simulink model "H8_6GDL_lineal_modelo"  (R2022b)
settings: Solver=VariableStepAuto  StartTime=0.0  StopTime=5  MaxStep=1e-3  RelTol=1e-3
InitFcn:
  | cg_nom=0.567;
  | cg_suelo=0.56985;
  | cg_techo=0.54735;
values from neighbouring files (symbols this model uses):
  A6 = [0 0 0 0 0 0 0 0 0 0 0 0 ... (100 elements, 10x10)]    [matrices_linealizacion_6gdl.mat]
  B6 = [0 0 0 0 0 0.000575563603666 -0.0459993641186 -0.0505103975277 0.151580453785 0.00175830093621 0 0 ... (80 elements, 10x8)]    [matrices_linealizacion_6gdl.mat]
  C6 = [1 0 0 0 0 0 0 0 0 0 0 1 ... (100 elements, 10x10)]    [matrices_linealizacion_6gdl.mat]
  D6 = [0 0 0 0 0 0 0 0 0 0 0 0 ... (80 elements, 10x8)]    [matrices_linealizacion_6gdl.mat]
  Ka = [34.5916764023 4.46928641015 34.7816336405 4.65924364837 92.2484067139 -92.2484067139 74.2332308826 -74.2332308826 -4220.94514487 -4209.6309051 -4205.06787146 -4193.7536317 ... (120 elements, 8x15)]    [Ka.mat]    (also in linealizacion_5gdl_bien.m = place(Aa,Ba,[ -1.5 -1.5 -1.5 -1.5 -2 -2 -6 -6 -7 -7 -5 -5 -2; linealizacion_EMS.m = place(Aa,Ba,[ -1 -1 -2 -2 -3 -3 -6 -6 -7 -7 -5 -5 -4 -4 -5 -)
undefined symbols (not defined in the file or in its folder): ems, hems, magnitude
libraries: simulink x5
settings Model: Creator=aceao  LastModifiedBy=USUARIO
settings SolverCC: ZeroCrossAlgorithm=Adaptive
settings DebuggingCC: IgnoredZcDiagnostic=none

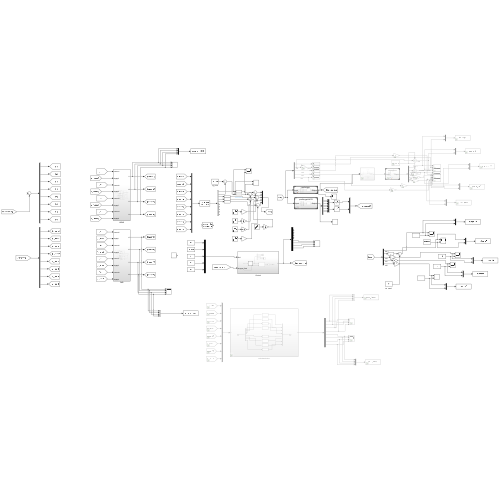
[thumbnail: Simulink's stored preview of the top-level diagram]
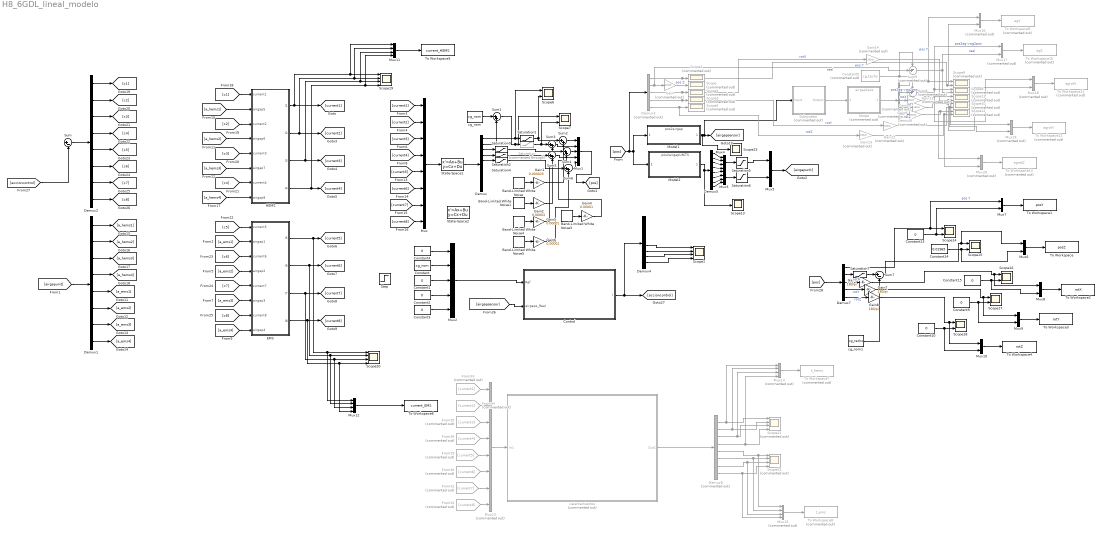
== system H8_6GDL_lineal_modelo ==
  Band-Limited White Noise : simulink/Sources/Band-Limited White Noise  Cov=[0.001]  Ts=0.1  seed=[1]
  Band-Limited White Noise1 : simulink/Sources/Band-Limited White Noise  Cov=[0.001]  Ts=0.1  seed=[2]
  Band-Limited White Noise3 : simulink/Sources/Band-Limited White Noise  Cov=[0.001]  Ts=0.1  seed=[4]
  Band-Limited White Noise4 : simulink/Sources/Band-Limited White Noise  Cov=[0.001]  Ts=0.1  seed=[3]
  Band-Limited White Noise5 : simulink/Sources/Band-Limited White Noise  Cov=[0.001]  Ts=0.1  seed=[5]
  Constant : Constant  Value=cg_nom
  Constant{1..4,9..10,13,15} (8 alike) : Constant  Value=0
  Constant14 : Constant  Value=0.01965
  Constant5 : Constant  Commented=on  Value=cg_techo
  Control : Subsystem
  Demux : Demux  Outputs=10
  Demux{1..2,4..5} (4 alike) : Demux  Outputs=8
  Demux3 : Demux  Commented=on  Outputs=5
  Demux6 : Demux  Commented=on  Outputs=5
  Demux7 : Demux  Outputs=5
  Demux8 : Demux  Commented=on  Outputs=8
  EMS : Subsystem
  From29 : From  Commented=on  GotoTag=current5
  From30 : From  Commented=on  GotoTag=current6
  From31 : From  Commented=on  GotoTag=current7
  From32 : From  Commented=on  GotoTag=current8
  From33 : From  Commented=on  GotoTag=current1
  From34 : From  Commented=on  GotoTag=current2
  From35 : From  Commented=on  GotoTag=current3
  From36 : From  Commented=on  GotoTag=current4
  Gain : Gain  Commented=on  Gain=1000
  Gain1 : Gain  Gain=0.000025
  Gain{9..14} (6 alike) : Gain  Commented=on  Gain=180/pi
  Gain2 : Gain  Gain=0.00003
  Gain3 : Gain  Gain=180/pi
  Gain4 : Gain  Gain=0.00001
  Gain5 : Gain  Gain=0.00001
  Gain6 : Gain  Gain=0.00001
  Gain7 : Gain  Gain=180/pi
  Gain8 : Gain  Gain=180/pi
  HEMS : Subsystem
  Model : ModelReference  Commented=on  ModelNameDialog=airgap2pos.slx  SimulationMode=Normal  ModelReferenceVersion=1.6
  Model1 : ModelReference  ModelNameDialog=pos2airgap.slx  SimulationMode=Normal  ModelReferenceVersion=1.6
  Model2 : ModelReference  ModelNameDialog=pos2airgapUNITS.slx  SimulationMode=Normal  ModelReferenceVersion=1.3
  Mux : Mux  Inputs=8
  Mux1 : Mux  Inputs=5
  Mux{5..10} (6 alike) : Mux  Inputs=2
  Mux{3..4,11..12} (4 alike) : Mux
  Mux13 : Mux  Commented=on  Inputs=8
  Mux14 : Mux  Commented=on
  Mux15 : Mux  Commented=on
  Mux{16..20} (5 alike) : Mux  Commented=on  Inputs=2
  Mux2 : Mux  Inputs=5
  Saturation : Saturate  Commented=through  UpperLimit=cg_suelo  LowerLimit=cg_techo
  Saturation1 : Saturate  UpperLimit=0.012  LowerLimit=-0.012
  Saturation2 : Saturate  UpperLimit=0.01268  LowerLimit=-0.01268
  Saturation3 : Saturate  UpperLimit=0.0476  LowerLimit=-0.0476
  Saturation4 : Saturate  UpperLimit=0.024  LowerLimit=-0.024
  Saturation5 : Saturate  UpperLimit=0.0225  LowerLimit=0.01
  Saturation6 : Saturate  UpperLimit=0.012  LowerLimit=-0.012
  Saturation7 : Saturate  UpperLimit=cg_suelo  LowerLimit=cg_techo
  Scope{,2..5} (5 alike) : Scope  Commented=on
  Scope1 : Scope  NumInputPorts=4
  Scope{8..12} (5 alike) : Scope  Commented=on  NumInputPorts=2
  Scope13 : Scope
  Scope{6..7,14..18} (7 alike) : Scope  NumInputPorts=2
  Scope19 : Scope  NumInputPorts=4
  Scope20 : Scope  NumInputPorts=4
  Scope21 : Scope  Commented=on  NumInputPorts=4
  Scope22 : Scope  Commented=on  NumInputPorts=4
  Scope23 : Scope
  State-Space1 : StateSpace  A=A6  B=B6  C=C6  D=D6  InitialCondition=[-0.002, +0.002, -0.001, 0.001, 0.001, 0, 0, 0, 0, 0]
  State-Space2 : StateSpace  A=A6  B=B6  C=C6  D=D6  InitialCondition=[ 0, cg_suelo-cg_nom, 0, 0, 0, 0, 0, 0, 0, 0]
  Step : Step  Time=0.25  Before=cg_suelo  After=cg_nom  SampleTime=0
  Subsystem : Subsystem  Commented=on
  Sum : Sum  Inputs=|+-
  Sum{1..6} (6 alike) : Sum  Inputs=|++
  Sum7 : Sum  Inputs=|+-
  Sum8 : Sum  Commented=on  Inputs=-+|
  Sum9 : Sum  Commented=on  Inputs=-+|
  To Workspace : ToWorkspace  VariableName=posZ  SaveFormat=Timeseries  SampleTime=-1
  To Workspace1 : ToWorkspace  VariableName=posY  SaveFormat=Timeseries  SampleTime=-1
  To Workspace10 : ToWorkspace  Commented=on  VariableName=agZ  SaveFormat=Timeseries  SampleTime=-1
  To Workspace11 : ToWorkspace  Commented=on  VariableName=agrotX  SaveFormat=Timeseries  SampleTime=-1
  To Workspace12 : ToWorkspace  Commented=on  VariableName=agrotY  SaveFormat=Timeseries  SampleTime=-1
  To Workspace13 : ToWorkspace  Commented=on  VariableName=agrotZ  SaveFormat=Timeseries  SampleTime=-1
  To Workspace2 : ToWorkspace  VariableName=rotX  SaveFormat=Timeseries  SampleTime=-1
  To Workspace3 : ToWorkspace  VariableName=rotY  SaveFormat=Timeseries  SampleTime=-1
  To Workspace4 : ToWorkspace  VariableName=rotZ  SaveFormat=Timeseries  SampleTime=-1
  To Workspace5 : ToWorkspace  VariableName=current_HEMS  SaveFormat=Timeseries  SampleTime=-1
  To Workspace6 : ToWorkspace  VariableName=current_EMS  SaveFormat=Timeseries  SampleTime=-1
  To Workspace7 : ToWorkspace  Commented=on  VariableName=t_hems  SaveFormat=Timeseries  SampleTime=-1
  To Workspace8 : ToWorkspace  Commented=on  VariableName=t_ems  SaveFormat=Timeseries  SampleTime=-1
  To Workspace9 : ToWorkspace  Commented=on  VariableName=agY  SaveFormat=Timeseries  SampleTime=-1
  calentamientos : Subsystem  Commented=on
  cg_nom : Constant  Value=cg_nom
  cg_nom1 : Constant  Value=cg_techo
  wires:
  Mux/1 -> State-Space1/1
  Demux/1 -> Scope6/1, Saturation1/1
  Mux1/1 -> [pos]
  [pos] -> Demux3/1, Model1/1, Model2/1
  Model2/1 -> Scope13/1, Demux5/1
  [current1] -> Mux/1
  [current2] -> Mux/2
  [current3] -> Mux/3
  [current4] -> Mux/4
  [current5] -> Mux/5
  [current6] -> Mux/6
  [current7] -> Mux/7
  [current8] -> Mux/8
  Model1/1 -> Scope23/1, Subsystem/1(Input), [airgapsensor]
  [airgapunit] -> Demux1/1
  [a_ems2] -> EMS/4(airgap2)
  [a_ems1] -> EMS/2(airgap1)
  [a_ems3] -> EMS/6(airgap3)
  [a_ems4] -> EMS/8(airgap4)
  [a_hems1] -> HEMS/2(airgap5)
  [a_hems2] -> HEMS/4(airgap6)
  [a_hems3] -> HEMS/6(airgap7)
  [a_hems4] -> HEMS/8(airgap8)
  Demux2/3 -> [c3]
  Demux2/1 -> [c1]
  Demux2/8 -> [c8]
  Demux2/5 -> [c5]
  Sum/1 -> Demux2/1
  Demux2/4 -> [c4]
  Demux2/6 -> [c6]
  Demux2/7 -> [c7]
  Demux2/2 -> [c2]
  [c1] -> HEMS/1(current1)
  [c2] -> HEMS/3(current2)
  [c3] -> HEMS/5(current3)
  [c4] -> HEMS/7(current4)
  [c5] -> EMS/1(current5)
  [c6] -> EMS/3(current6)
  [c7] -> EMS/5(current7)
  [c8] -> EMS/7(current8)
  Demux/2 -> Sum1/2
  Sum1/1 -> Scope7/1, Saturation/1
  cg_nom/1 -> Sum1/1
  Control/1(I) -> Demux4/1, [accioncontrol]
  [airgapsensor] -> Control/2(airgaps_Real)
  [accioncontrol] -> Sum/2
  Mux2/1 -> Control/1(Ref)
  Constant1/1 -> Mux2/3
  Constant2/1 -> Mux2/4
  Constant3/1 -> Mux2/5
  Constant4/1 -> Mux2/1
  Demux3/2 -> Sum9/2, Gain/1  "real"
  Demux4/5 -> Scope1/1
  Demux4/6 -> Scope1/2
  Demux4/7 -> Scope1/3
  Demux4/8 -> Scope1/4
  Demux3/1 -> Mux16/2, Scope9/2, Scope2/1  "pos Y"
  Demux3/3 -> Gain14/1, Scope4/1  "rotX"
  Demux3/4 -> Gain12/1, Scope3/1  "rotY"
  Demux3/5 -> Gain13/1, Scope5/1  "rotZ"
  Gain/1 -> Scope/1  "pos Z"
  Saturation/1 -> Sum3/1, Scope7/2
  Demux/3 -> Saturation3/1
  Demux/4 -> Saturation2/1
  Demux/5 -> Saturation4/1
  Demux5/1 -> Mux4/1
  Demux5/2 -> Mux4/2
  Demux5/3 -> Mux4/3
  Demux5/4 -> Mux4/4
  Demux5/5 -> Mux3/1
  Demux5/6 -> Mux3/2
  Demux5/7 -> Mux3/3
  Demux5/8 -> Mux3/4
  Mux4/1 -> Saturation5/1
  Mux5/1 -> [airgapunit]
  Saturation5/1 -> Mux5/1
  Mux3/1 -> Saturation6/1
  Saturation6/1 -> Mux5/2
  Demux1/2 -> [a_hems2]
  Demux1/3 -> [a_hems3]
  Demux1/4 -> [a_hems4]
  Demux1/1 -> [a_hems1]
  Demux1/5 -> [a_ems1]
  Demux1/7 -> [a_ems3]
  Demux1/6 -> [a_ems2]
  Demux1/8 -> [a_ems4]
  Saturation3/1 -> Sum4/1
  Saturation2/1 -> Sum5/1
  Saturation4/1 -> Sum6/1
  Saturation1/1 -> Scope6/2, Sum2/1
  State-Space1/1 -> Demux/1
  HEMS/1(I1) -> Mux11/1, Scope19/1, [current1]
  HEMS/2(I2) -> Mux11/2, Scope19/2, [current2]
  HEMS/4(I4) -> Mux11/4, Scope19/4, [current4]
  HEMS/3(I3) -> Mux11/3, Scope19/3, [current3]
  Model/1 -> Demux6/1
  Demux6/5 -> Gain9/1  "rotZ"
  Demux6/1 -> Mux16/1, Scope9/1  "pos Y"
  Demux6/3 -> Gain11/1  "rotX"
  Sum8/1 -> Mux17/1, Scope8/1  "pos2ag->ag2pos"
  Demux6/4 -> Gain10/1  "rotY"
  Sum2/1 -> Mux1/1
  Sum3/1 -> Mux1/2
  Sum4/1 -> Mux1/3
  Sum5/1 -> Mux1/4
  Sum6/1 -> Mux1/5
  Band-Limited White Noise1/1 -> Gain2/1
  Band-Limited White Noise/1 -> Gain1/1
  Band-Limited White Noise3/1 -> Gain4/1
  Band-Limited White Noise4/1 -> Gain5/1
  Band-Limited White Noise5/1 -> Gain6/1
  Gain1/1 -> Sum2/2
  Gain2/1 -> Sum3/2
  Gain5/1 -> Sum5/2
  Gain4/1 -> Sum4/2
  Gain6/1 -> Sum6/2
  [pos] -> Demux7/1
  Demux7/2 -> Saturation7/1
  cg_nom1/1 -> Sum7/2
  Demux7/3 -> Gain3/1  "rotX"
  Demux7/4 -> Gain7/1  "rotY"
  Demux7/5 -> Gain8/1  "rotZ"
  Gain8/1 -> Mux10/1, Scope18/1
  Gain7/1 -> Mux9/1, Scope17/1
  Gain3/1 -> Mux8/1, Scope16/1
  Constant13/1 -> Mux7/2, Scope14/2
  Sum7/1 -> Mux6/1, Scope15/1
  Demux7/1 -> Mux7/1, Scope14/1  "pos Y"
  Constant14/1 -> Mux6/2, Scope15/2
  Constant15/1 -> Mux8/2, Scope16/2
  Constant9/1 -> Mux9/2, Scope17/2
  Constant10/1 -> Mux10/2, Scope18/2
  Mux6/1 -> To Workspace/1
  Constant/1 -> Mux2/2
  Saturation7/1 -> Sum7/1
  Mux7/1 -> To Workspace1/1
  Mux8/1 -> To Workspace2/1
  Mux9/1 -> To Workspace3/1
  Mux10/1 -> To Workspace4/1
  Mux11/1 -> To Workspace5/1
  Mux12/1 -> To Workspace6/1
  EMS/3(I7) -> [current7], Mux12/3, Scope20/3
  EMS/2(I6) -> [current6], Mux12/2, Scope20/2
  EMS/4(I8) -> Mux12/4, Scope20/4, [current8]
  From34/1 -> Mux13/2
  From33/1 -> Mux13/1
  From29/1 -> Mux13/5
  From30/1 -> Mux13/6
  From36/1 -> Mux13/4
  Mux13/1 -> calentamientos/1(In1)
  From35/1 -> Mux13/3
  From31/1 -> Mux13/7
  From32/1 -> Mux13/8
  calentamientos/1(Out1) -> Demux8/1
  Demux8/1 -> Mux14/1, Scope21/1
  Demux8/2 -> Mux14/2, Scope21/2
  Demux8/3 -> Scope21/3, Mux14/3
  Demux8/4 -> Scope21/4, Mux14/4
  Mux14/1 -> To Workspace7/1
  EMS/1(I5) -> Mux12/1, Scope20/1, [current5]
  Demux8/5 -> Mux15/1, Scope22/1
  Demux8/6 -> Mux15/2, Scope22/2
  Demux8/7 -> Mux15/3, Scope22/3
  Demux8/8 -> Mux15/4, Scope22/4
  Mux15/1 -> To Workspace8/1
  Subsystem/1(Output) -> Model/1
  Mux16/1 -> To Workspace9/1
  Mux17/1 -> To Workspace10/1
  Mux18/1 -> To Workspace11/1
  Mux19/1 -> To Workspace12/1
  Mux20/1 -> To Workspace13/1
  Gain11/1 -> Mux18/1, Scope11/1
  Gain10/1 -> Mux19/1, Scope10/1
  Gain9/1 -> Scope12/1, Mux20/1
  Gain12/1 -> Mux19/2, Scope10/2
  Gain13/1 -> Mux20/2, Scope12/2
  Gain14/1 -> Mux18/2, Scope11/2
  Demux6/2 -> Sum8/2  "pos2ag->ag2pos"
  Constant5/1 -> Sum9/1, Sum8/1
  Sum9/1 -> Scope8/2, Mux17/2  "real"

== system H8_6GDL_lineal_modelo/Control ==
  Ref : Inport
  airgaps_Real : Inport  Port=2
  Demux : Demux  Outputs=5
  Model : ModelReference  ModelNameDialog=airgap2pos.slx  SimulationMode=Normal  ModelReferenceVersion=1.6
  Saturation4 : Saturate  Commented=through  UpperLimit=55  LowerLimit=-55
  Scope : Scope  NumInputPorts=3
  Scope1 : Scope  NumInputPorts=2
  state space control : Subsystem
  I : Outport
  wires:
  airgaps_Real/1 -> Model/1
  Saturation4/1 -> I/1
  Model/1 -> Demux/1, state space control/1(In1)
  Ref/1 -> state space control/2(In2)
  state space control/1(Out1) -> Saturation4/1
  Demux/1 -> Scope1/1
  Demux/3 -> Scope/1
  Demux/4 -> Scope/2
  Demux/5 -> Scope/3
  Demux/2 -> Scope1/2

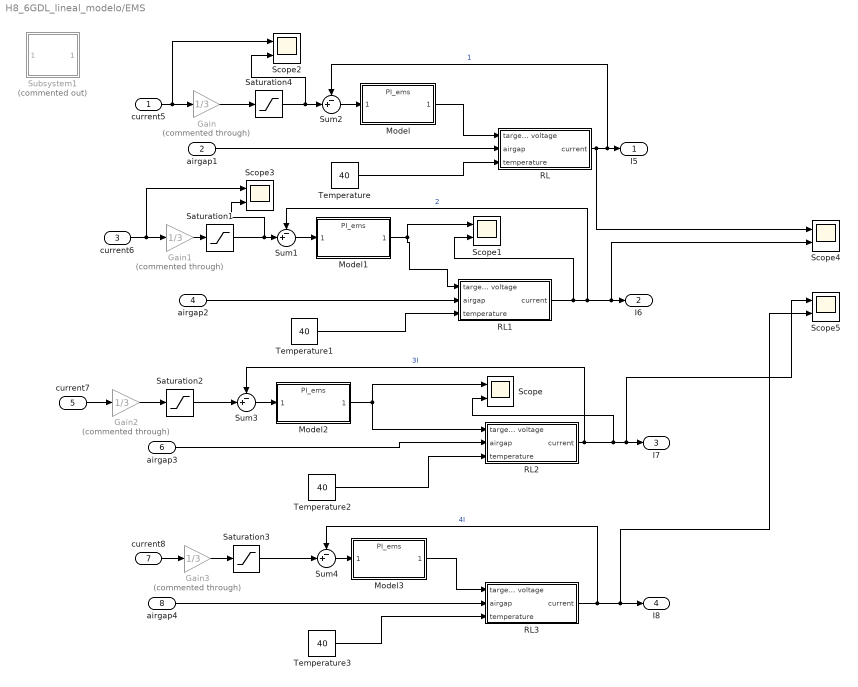
== system H8_6GDL_lineal_modelo/EMS ==
  current5 : Inport
  airgap1 : Inport  Port=2
  current6 : Inport  Port=3
  airgap2 : Inport  Port=4
  current7 : Inport  Port=5
  airgap3 : Inport  Port=6
  current8 : Inport  Port=7
  airgap4 : Inport  Port=8
  Gain{,1..3} (4 alike) : Gain  Commented=through  Gain=1/3
  Model{,1..3} (4 alike) : ModelReference  ModelNameDialog=PI_ems.slx  SimulationMode=Normal  ModelReferenceVersion=1.2
  RL : Subsystem
  RL1 : Subsystem
  RL2 : Subsystem
  RL3 : Subsystem
  Saturation{1..4} (4 alike) : Saturate  UpperLimit=50  LowerLimit=0
  Scope{,1..5} (6 alike) : Scope  NumInputPorts=2
  Subsystem1 : Subsystem  Commented=on
  Sum{1..4} (4 alike) : Sum  Inputs=-+|
  Temperature{,1..3} (4 alike) : Constant  Value=40
  I5 : Outport
  I6 : Outport  Port=2
  I7 : Outport  Port=3
  I8 : Outport  Port=4
  wires:
  Temperature/1 -> RL/3(temperature)
  airgap1/1 -> RL/2(airgap)
  Temperature3/1 -> RL3/3(temperature)
  RL/1(current) -> Scope4/1, I5/1, Sum2/1  "1"
  current8/1 -> Gain3/1
  Temperature1/1 -> RL1/3(temperature)
  Temperature2/1 -> RL2/3(temperature)
  RL3/1(current) -> Scope5/2, I8/1, Sum4/1  "4I"
  current7/1 -> Gain2/1
  airgap2/1 -> RL1/2(airgap)
  RL1/1(current) -> Scope1/2, Scope4/2, I6/1, Sum1/1  "2"
  RL2/1(current) -> Scope/2, Scope5/1, I7/1, Sum3/1  "3I"
  airgap3/1 -> RL2/2(airgap)
  airgap4/1 -> RL3/2(airgap)
  Sum2/1 -> Model/1
  Sum1/1 -> Model1/1
  Sum3/1 -> Model2/1
  Sum4/1 -> Model3/1
  Model/1 -> RL/1(target voltage)
  Model3/1 -> RL3/1(target voltage)
  Model2/1 -> RL2/1(target voltage), Scope/1
  Model1/1 -> RL1/1(target voltage), Scope1/1
  current5/1 -> Scope2/1, Gain/1
  Saturation4/1 -> Scope2/2, Sum2/2
  Saturation1/1 -> Scope3/2, Sum1/2
  Saturation2/1 -> Sum3/2
  Saturation3/1 -> Sum4/2
  current6/1 -> Scope3/1, Gain1/1
  Gain/1 -> Saturation4/1
  Gain1/1 -> Saturation1/1
  Gain2/1 -> Saturation2/1
  Gain3/1 -> Saturation3/1

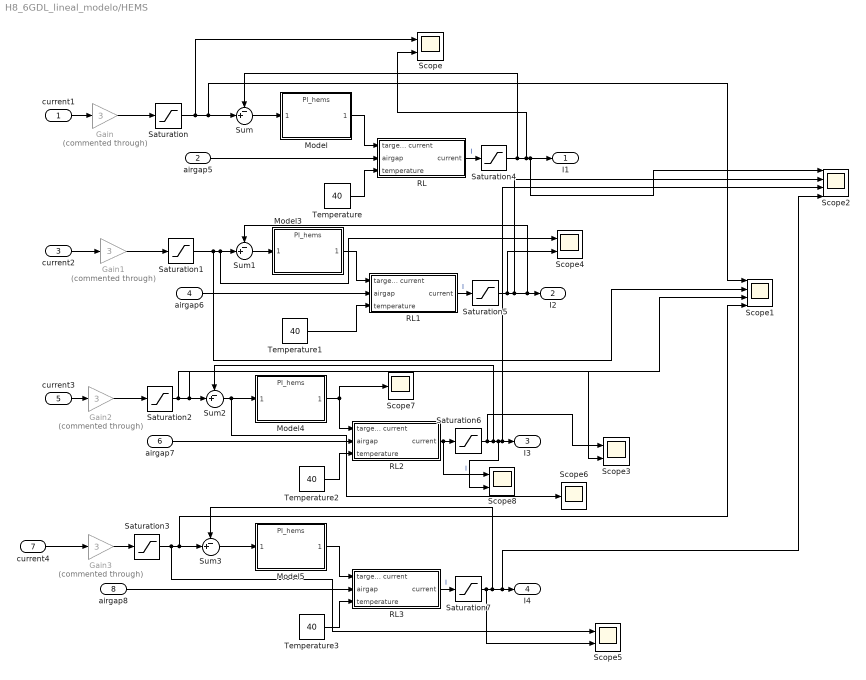
== system H8_6GDL_lineal_modelo/HEMS ==
  current1 : Inport
  airgap5 : Inport  Port=2
  current2 : Inport  Port=3
  airgap6 : Inport  Port=4
  current3 : Inport  Port=5
  airgap7 : Inport  Port=6
  current4 : Inport  Port=7
  airgap8 : Inport  Port=8
  Gain{,1..3} (4 alike) : Gain  Commented=through  Gain=3
  Model{,3..5} (4 alike) : ModelReference  ModelNameDialog=PI_hems.slx  SimulationMode=Normal  ModelReferenceVersion=1.3
  RL : Subsystem
  RL1 : Subsystem
  RL2 : Subsystem
  RL3 : Subsystem
  Saturation{,1..7} (8 alike) : Saturate  UpperLimit=50  LowerLimit=-50
  Scope{,3..5,8} (5 alike) : Scope  NumInputPorts=2
  Scope1 : Scope  NumInputPorts=4
  Scope2 : Scope  NumInputPorts=4
  Scope6 : Scope
  Scope7 : Scope
  Sum{,1..3} (4 alike) : Sum  Inputs=-+|
  Temperature{,1..3} (4 alike) : Constant  Value=40
  I1 : Outport
  I2 : Outport  Port=2
  I3 : Outport  Port=3
  I4 : Outport  Port=4
  wires:
  Temperature/1 -> RL/3(temperature)
  Model3/1 -> RL1/1(target current)
  Model5/1 -> RL3/1(target current)
  Model/1 -> RL/1(target current)
  airgap5/1 -> RL/2(airgap)
  Temperature3/1 -> RL3/3(temperature)
  RL/1(current) -> Saturation4/1  "I"
  current4/1 -> Gain3/1
  Temperature1/1 -> RL1/3(temperature)
  Temperature2/1 -> RL2/3(temperature)
  Model4/1 -> RL2/1(target current), Scope7/1
  RL3/1(current) -> Saturation7/1  "I"
  current3/1 -> Gain2/1
  current1/1 -> Gain/1
  airgap6/1 -> RL1/2(airgap)
  RL1/1(current) -> Saturation5/1  "I"
  current2/1 -> Gain1/1
  RL2/1(current) -> Scope8/1, Saturation6/1  "I"
  airgap7/1 -> RL2/2(airgap)
  airgap8/1 -> RL3/2(airgap)
  Sum/1 -> Model/1
  Sum1/1 -> Model3/1
  Sum2/1 -> Scope6/1, Model4/1
  Sum3/1 -> Model5/1
  Saturation2/1 -> Scope3/2, Scope1/3, Sum2/2
  Saturation1/1 -> Scope1/2, Scope4/1, Sum1/2
  Saturation/1 -> Scope/1, Scope1/1, Sum/2
  Saturation3/1 -> Scope5/1, Scope1/4, Sum3/2
  Gain/1 -> Saturation/1
  Gain3/1 -> Saturation3/1
  Gain2/1 -> Saturation2/1
  Gain1/1 -> Saturation1/1
  Saturation4/1 -> Scope/2, Scope2/1, I1/1, Sum/1
  Saturation5/1 -> Scope4/2, Scope2/2, Sum1/1, I2/1
  Saturation7/1 -> Scope5/2, Scope2/4, I4/1, Sum3/1
  Saturation6/1 -> Scope3/1, Scope8/2, Scope2/3, I3/1, Sum2/1

== system H8_6GDL_lineal_modelo/Subsystem ==
  Input : Inport
  Demux : Demux  Outputs=8
  Model{1..8} (8 alike) : ModelReference  ModelNameDialog=sensor_airgap.slx  SimulationMode=Normal  ModelReferenceVersion=1.3
  Mux : Mux  Inputs=8
  Scope{,1..3} (4 alike) : Scope  NumInputPorts=2
  Output : Outport
  wires:
  Demux/1 -> Model4/1, Scope/1
  Model4/1 -> Scope/2, Mux/1
  Model1/1 -> Mux/2, Scope1/2
  Demux/2 -> Model1/1, Scope1/1
  Model2/1 -> Scope2/2, Mux/3
  Demux/3 -> Model2/1, Scope2/1
  Model3/1 -> Mux/4
  Demux/4 -> Model3/1
  Model5/1 -> Scope3/2, Mux/5
  Demux/5 -> Model5/1, Scope3/1
  Model6/1 -> Mux/6
  Demux/6 -> Model6/1
  Model7/1 -> Mux/7
  Demux/7 -> Model7/1
  Model8/1 -> Mux/8
  Demux/8 -> Model8/1
  Input/1 -> Demux/1
  Mux/1 -> Output/1

== system H8_6GDL_lineal_modelo/calentamientos ==
  In1 : Inport
  Calentamiento 1 - bobina : Subsystem
  Calentamiento 1 - bobina1 : Subsystem
  Calentamiento 1 - bobina2 : Subsystem
  Calentamiento 1 - bobina3 : Subsystem
  Calentamiento 1 - bobina4 : Subsystem
  Calentamiento 1 - bobina5 : Subsystem
  Calentamiento 1 - bobina6 : Subsystem
  Calentamiento 1 - bobina7 : Subsystem
  Demux : Demux  Outputs=8
  Mux13 : Mux  Inputs=8
  Out1 : Outport
  wires:
  In1/1 -> Demux/1
  Demux/1 -> Calentamiento 1 - bobina/1(I (A))
  Demux/2 -> Calentamiento 1 - bobina1/1(I (A))
  Demux/3 -> Calentamiento 1 - bobina2/1(I (A))
  Demux/4 -> Calentamiento 1 - bobina3/1(I (A))
  Demux/5 -> Calentamiento 1 - bobina4/1(I (A))
  Demux/6 -> Calentamiento 1 - bobina5/1(I (A))
  Demux/7 -> Calentamiento 1 - bobina6/1(I (A))
  Demux/8 -> Calentamiento 1 - bobina7/1(I (A))
  Mux13/1 -> Out1/1
  Calentamiento 1 - bobina/1(T [ºC]) -> Mux13/1
  Calentamiento 1 - bobina1/1(T [ºC]) -> Mux13/2
  Calentamiento 1 - bobina2/1(T [ºC]) -> Mux13/3
  Calentamiento 1 - bobina3/1(T [ºC]) -> Mux13/4
  Calentamiento 1 - bobina4/1(T [ºC]) -> Mux13/5
  Calentamiento 1 - bobina5/1(T [ºC]) -> Mux13/6
  Calentamiento 1 - bobina6/1(T [ºC]) -> Mux13/7
  Calentamiento 1 - bobina7/1(T [ºC]) -> Mux13/8

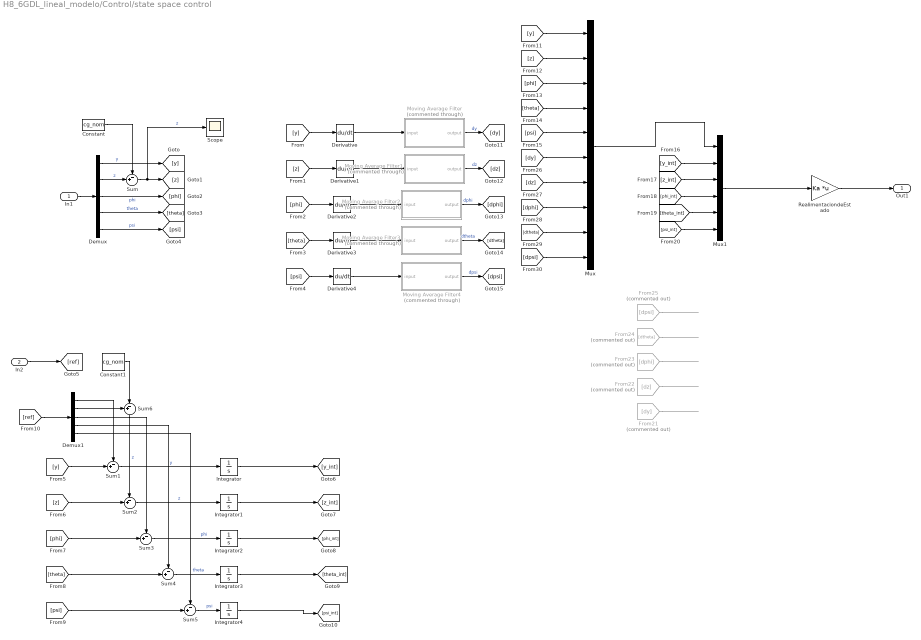
== system H8_6GDL_lineal_modelo/Control/state space control ==
  In1 : Inport
  In2 : Inport  Port=2
  Constant : Constant  Value=cg_nom
  Constant1 : Constant  Value=cg_nom
  Demux : Demux  Outputs=5
  Demux1 : Demux  Outputs=5
  Derivative{,1..4} (5 alike) : Derivative
  From21 : From  Commented=on  GotoTag=dy
  From22 : From  Commented=on  GotoTag=dz
  From23 : From  Commented=on  GotoTag=dphi
  From24 : From  Commented=on  GotoTag=dtheta
  From25 : From  Commented=on  GotoTag=dpsi
  Integrator{,1..4} (5 alike) : Integrator
  Moving Average Filter : Subsystem  Commented=through  mask{M=4, fs=-1}
      mask prompts: M "Orden del filtro (M)"; fs "Frecuencia de muestreo (fs)"
  Moving Average Filter1 : Subsystem  Commented=through  mask{M=4, fs=-1}
      mask prompts: M "Orden del filtro (M)"; fs "Frecuencia de muestreo (fs)"
  Moving Average Filter2 : Subsystem  Commented=through  mask{M=4, fs=-1}
      mask prompts: M "Orden del filtro (M)"; fs "Frecuencia de muestreo (fs)"
  Moving Average Filter3 : Subsystem  Commented=through  mask{M=4, fs=-1}
      mask prompts: M "Orden del filtro (M)"; fs "Frecuencia de muestreo (fs)"
  Moving Average Filter4 : Subsystem  Commented=through  mask{M=4, fs=-1}
      mask prompts: M "Orden del filtro (M)"; fs "Frecuencia de muestreo (fs)"
  Mux : Mux  Inputs=10
  Mux1 : Mux  Inputs=6
  RealimentaciondeEstado : Gain  Gain=Ka  Multiplication=Matrix(K*u)
  Scope : Scope
  Sum{,1..5} (6 alike) : Sum  Inputs=-+|
  Sum6 : Sum  Inputs=+-|
  Out1 : Outport
  wires:
  In1/1 -> Demux/1
  Derivative/1 -> Moving Average Filter/1(input)
  Derivative1/1 -> Moving Average Filter1/1(input)
  Derivative2/1 -> Moving Average Filter2/1(input)
  Derivative3/1 -> Moving Average Filter3/1(input)
  Derivative4/1 -> Moving Average Filter4/1(input)
  Demux/1 -> [y]  "y"
  Constant/1 -> Sum/1
  Sum/1 -> Scope/1, [z]  "z"
  Demux/2 -> Sum/2  "z"
  Demux/3 -> [phi]  "phi"
  Demux/4 -> [theta]  "theta"
  Demux/5 -> [psi]  "psi"
  [psi] -> Derivative4/1
  [theta] -> Derivative3/1
  [phi] -> Derivative2/1
  [z] -> Derivative1/1
  [y] -> Derivative/1
  In2/1 -> [ref]
  [ref] -> Demux1/1
  [y] -> Sum1/2
  [z] -> Sum2/2
  [phi] -> Sum3/2
  [theta] -> Sum4/2
  [psi] -> Sum5/2
  Demux1/1 -> Sum1/1
  Demux1/3 -> Sum3/1
  Demux1/4 -> Sum4/1
  Demux1/5 -> Sum5/1
  Sum1/1 -> Integrator/1  "y"
  Sum5/1 -> Integrator4/1  "psi"
  Sum4/1 -> Integrator3/1  "theta"
  Sum3/1 -> Integrator2/1  "phi"
  Sum2/1 -> Integrator1/1  "z"
  [y] -> Mux/1
  [z] -> Mux/2
  [phi] -> Mux/3
  [theta] -> Mux/4
  [psi] -> Mux/5
  Integrator/1 -> [y_int]
  Integrator1/1 -> [z_int]
  Integrator2/1 -> [phi_int]
  Integrator3/1 -> [theta_int]
  Moving Average Filter/1(output) -> [dy]  "dy"
  Moving Average Filter1/1(output) -> [dz]  "dz"
  Moving Average Filter2/1(output) -> [dphi]  "dphi"
  Moving Average Filter4/1(output) -> [dpsi]  "dpsi"
  Moving Average Filter3/1(output) -> [dtheta]  "dtheta"
  [y_int] -> Mux1/2
  [psi_int] -> Mux1/6
  [theta_int] -> Mux1/5
  [phi_int] -> Mux1/4
  [z_int] -> Mux1/3
  Constant1/1 -> Sum6/2
  Demux1/2 -> Sum6/1
  Sum6/1 -> Sum2/1  "z"
  Integrator4/1 -> [psi_int]
  [dtheta] -> Mux/9
  [dy] -> Mux/6
  [dz] -> Mux/7
  [dpsi] -> Mux/10
  [dphi] -> Mux/8
  From23/1 -> ?
  From24/1 -> ?
  From22/1 -> ?
  From21/1 -> ?
  From25/1 -> ?
  Mux1/1 -> RealimentaciondeEstado/1
  RealimentaciondeEstado/1 -> Out1/1
  Mux/1 -> Mux1/1

== system H8_6GDL_lineal_modelo/EMS/RL ==
  target voltage : Inport
  airgap : Inport  Port=2
  temperature : Inport  Port=3
  2-D Lookup Table : Lookup_n-D  BreakpointsForDimension1=ems.Airgap  BreakpointsForDimension2=ems.Flux_Current(2:55)  Table=ems.Inductance  InternalRulePriority=Speed  RndMeth=Simplest
      settings: InputPortMap=u0,u1
  Abs : Abs  SaturateOnIntegerOverflow=off
  Add : Sum  Inputs=+-
  Delay{,1..3} (4 alike) : Delay  DelayLength=1
  Divide : Product  Inputs=*/
  Divide1 : Product  Inputs=*/
  Divide2 : Product  Inputs=*/
  Integrator1 : Integrator
  Subsystem : Subsystem
  to mm : Gain  Gain=1000
  current : Outport
  wires:
  airgap/1 -> to mm/1
  Divide/1 -> Integrator1/1
  Add/1 -> Divide/1
  Integrator1/1 -> Abs/1, current/1, Delay3/1, Add/2  "current applied"
  2-D Lookup Table/1 -> Divide2/1  "L"
  target voltage/1 -> Divide1/1
  temperature/1 -> Delay2/1
  Divide1/1 -> Add/1
  Subsystem/1(R) -> Divide2/2, Divide1/2  "R"
  Delay3/1 -> Subsystem/1(Current)
  Delay2/1 -> Subsystem/2(Temperature)
  Divide2/1 -> Divide/2
  Delay1/1 -> 2-D Lookup Table/2
  Delay/1 -> 2-D Lookup Table/1
  Abs/1 -> Delay1/1
  to mm/1 -> Delay/1

== system H8_6GDL_lineal_modelo/EMS/RL1 ==
  target voltage : Inport
  airgap : Inport  Port=2
  temperature : Inport  Port=3
  2-D Lookup Table : Lookup_n-D  BreakpointsForDimension1=ems.Airgap  BreakpointsForDimension2=ems.Flux_Current(2:55)  Table=ems.Inductance  InternalRulePriority=Speed  RndMeth=Simplest
      settings: InputPortMap=u0,u1
  Abs : Abs  SaturateOnIntegerOverflow=off
  Add : Sum  Inputs=+-
  Delay{,1..3} (4 alike) : Delay  DelayLength=1
  Divide : Product  Inputs=*/
  Divide1 : Product  Inputs=*/
  Divide2 : Product  Inputs=*/
  Integrator1 : Integrator
  Subsystem : Subsystem
  to mm : Gain  Gain=1000
  current : Outport
  wires:
  airgap/1 -> to mm/1
  Divide/1 -> Integrator1/1
  Add/1 -> Divide/1
  Integrator1/1 -> Abs/1, current/1, Delay3/1, Add/2  "current applied"
  2-D Lookup Table/1 -> Divide2/1  "L"
  target voltage/1 -> Divide1/1
  temperature/1 -> Delay2/1
  Divide1/1 -> Add/1
  Subsystem/1(R) -> Divide2/2, Divide1/2  "R"
  Delay3/1 -> Subsystem/1(Current)
  Delay2/1 -> Subsystem/2(Temperature)
  Divide2/1 -> Divide/2
  Delay1/1 -> 2-D Lookup Table/2
  Delay/1 -> 2-D Lookup Table/1
  Abs/1 -> Delay1/1
  to mm/1 -> Delay/1

== system H8_6GDL_lineal_modelo/EMS/RL2 ==
  target voltage : Inport
  airgap : Inport  Port=2
  temperature : Inport  Port=3
  2-D Lookup Table : Lookup_n-D  BreakpointsForDimension1=ems.Airgap  BreakpointsForDimension2=ems.Flux_Current(2:55)  Table=ems.Inductance  InternalRulePriority=Speed  RndMeth=Simplest
      settings: InputPortMap=u0,u1
  Abs : Abs  SaturateOnIntegerOverflow=off
  Add : Sum  Inputs=+-
  Delay{,1..3} (4 alike) : Delay  DelayLength=1
  Divide : Product  Inputs=*/
  Divide1 : Product  Inputs=*/
  Divide2 : Product  Inputs=*/
  Integrator1 : Integrator
  Subsystem : Subsystem
  to mm : Gain  Gain=1000
  current : Outport
  wires:
  airgap/1 -> to mm/1
  Divide/1 -> Integrator1/1
  Add/1 -> Divide/1
  Integrator1/1 -> Abs/1, current/1, Delay3/1, Add/2  "current applied"
  2-D Lookup Table/1 -> Divide2/1  "L"
  target voltage/1 -> Divide1/1
  temperature/1 -> Delay2/1
  Divide1/1 -> Add/1
  Subsystem/1(R) -> Divide2/2, Divide1/2  "R"
  Delay3/1 -> Subsystem/1(Current)
  Delay2/1 -> Subsystem/2(Temperature)
  Divide2/1 -> Divide/2
  Delay1/1 -> 2-D Lookup Table/2
  Delay/1 -> 2-D Lookup Table/1
  Abs/1 -> Delay1/1
  to mm/1 -> Delay/1

== system H8_6GDL_lineal_modelo/EMS/RL3 ==
  target voltage : Inport
  airgap : Inport  Port=2
  temperature : Inport  Port=3
  2-D Lookup Table : Lookup_n-D  BreakpointsForDimension1=ems.Airgap  BreakpointsForDimension2=ems.Flux_Current(2:55)  Table=ems.Inductance  InternalRulePriority=Speed  RndMeth=Simplest
      settings: InputPortMap=u0,u1
  Abs : Abs  SaturateOnIntegerOverflow=off
  Add : Sum  Inputs=+-
  Delay{,1..3} (4 alike) : Delay  DelayLength=1
  Divide : Product  Inputs=*/
  Divide1 : Product  Inputs=*/
  Divide2 : Product  Inputs=*/
  Integrator1 : Integrator
  Subsystem : Subsystem
  to mm : Gain  Gain=1000
  current : Outport
  wires:
  airgap/1 -> to mm/1
  Divide/1 -> Integrator1/1
  Add/1 -> Divide/1
  Integrator1/1 -> Abs/1, current/1, Delay3/1, Add/2  "current applied"
  2-D Lookup Table/1 -> Divide2/1  "L"
  target voltage/1 -> Divide1/1
  temperature/1 -> Delay2/1
  Divide1/1 -> Add/1
  Subsystem/1(R) -> Divide2/2, Divide1/2  "R"
  Delay3/1 -> Subsystem/1(Current)
  Delay2/1 -> Subsystem/2(Temperature)
  Divide2/1 -> Divide/2
  Delay1/1 -> 2-D Lookup Table/2
  Delay/1 -> 2-D Lookup Table/1
  Abs/1 -> Delay1/1
  to mm/1 -> Delay/1

== system H8_6GDL_lineal_modelo/EMS/Subsystem1 ==
  current5 : Inport
  Constant : Constant  Value=0
  Constant2 : Constant  Value=50
  Switch : Switch  Criteria=u2 > Threshold  SaturateOnIntegerOverflow=off  InputSameDT=off
  Switch1 : Switch  Criteria=u2 > Threshold  Threshold=50  SaturateOnIntegerOverflow=off  InputSameDT=off
  Out1 : Outport
  wires:
  current5/1 -> Switch/1, Switch/2
  Switch1/1 -> Out1/1
  Switch/1 -> Switch1/3, Switch1/2
  Constant/1 -> Switch/3
  Constant2/1 -> Switch1/1

== system H8_6GDL_lineal_modelo/HEMS/RL ==
  target current : Inport
  airgap : Inport  Port=2
  temperature : Inport  Port=3
  2-D Lookup Table : Lookup_n-D  BreakpointsForDimension1=hems.Airgap  BreakpointsForDimension2=hems.Current(2:110)  Table=hems.Inductance  InternalRulePriority=Speed  RndMeth=Simplest
      settings: InputPortMap=u0,u1
  Add : Sum  Inputs=+-
  Delay{1..4} (4 alike) : Delay  DelayLength=1
  Divide : Product  Inputs=*/
  Divide1 : Product  Inputs=*/
  Divide2 : Product  Inputs=*/
  Integrator1 : Integrator
  Rate Transition : RateTransition  Commented=through
  Saturation5 : Saturate  UpperLimit=0.0225  LowerLimit=0.01
  Subsystem : Subsystem
  to mm : Gain  Gain=1000
  current : Outport
  wires:
  airgap/1 -> Saturation5/1
  Divide/1 -> Integrator1/1
  Add/1 -> Divide/1
  Integrator1/1 -> Delay1/1, current/1, Delay3/1, Add/2  "current applied"
  2-D Lookup Table/1 -> Divide2/1  "L"
  target current/1 -> Divide1/1
  temperature/1 -> Delay2/1
  Divide1/1 -> Add/1
  Subsystem/1(R) -> Divide2/2, Divide1/2  "R"
  Delay3/1 -> Subsystem/1(Current)
  Delay2/1 -> Subsystem/2(Temperature)
  Divide2/1 -> Divide/2
  Delay1/1 -> 2-D Lookup Table/2
  Rate Transition/1 -> 2-D Lookup Table/1
  Saturation5/1 -> to mm/1
  to mm/1 -> Delay4/1
  Delay4/1 -> Rate Transition/1

== system H8_6GDL_lineal_modelo/HEMS/RL1 ==
  target current : Inport
  airgap : Inport  Port=2
  temperature : Inport  Port=3
  2-D Lookup Table : Lookup_n-D  BreakpointsForDimension1=hems.Airgap  BreakpointsForDimension2=hems.Current(2:110)  Table=hems.Inductance  InternalRulePriority=Speed  RndMeth=Simplest
      settings: InputPortMap=u0,u1
  Add : Sum  Inputs=+-
  Delay{1..4} (4 alike) : Delay  DelayLength=1
  Divide : Product  Inputs=*/
  Divide1 : Product  Inputs=*/
  Divide2 : Product  Inputs=*/
  Integrator1 : Integrator
  Rate Transition : RateTransition  Commented=through
  Saturation1 : Saturate  UpperLimit=0.0225  LowerLimit=0.01
  Subsystem : Subsystem
  to mm : Gain  Gain=1000
  current : Outport
  wires:
  airgap/1 -> Saturation1/1
  Divide/1 -> Integrator1/1
  Add/1 -> Divide/1
  Integrator1/1 -> Delay1/1, current/1, Delay3/1, Add/2  "current applied"
  2-D Lookup Table/1 -> Divide2/1  "L"
  target current/1 -> Divide1/1
  temperature/1 -> Delay2/1
  Divide1/1 -> Add/1
  Subsystem/1(R) -> Divide2/2, Divide1/2  "R"
  Delay3/1 -> Subsystem/1(Current)
  Delay2/1 -> Subsystem/2(Temperature)
  Divide2/1 -> Divide/2
  Delay1/1 -> 2-D Lookup Table/2
  Rate Transition/1 -> 2-D Lookup Table/1
  Saturation1/1 -> to mm/1
  to mm/1 -> Delay4/1
  Delay4/1 -> Rate Transition/1

== system H8_6GDL_lineal_modelo/HEMS/RL2 ==
  target current : Inport
  airgap : Inport  Port=2
  temperature : Inport  Port=3
  2-D Lookup Table : Lookup_n-D  BreakpointsForDimension1=hems.Airgap  BreakpointsForDimension2=hems.Current(2:110)  Table=hems.Inductance  InternalRulePriority=Speed  RndMeth=Simplest
      settings: InputPortMap=u0,u1
  Add : Sum  Inputs=+-
  Delay{1..4} (4 alike) : Delay  DelayLength=1
  Divide : Product  Inputs=*/
  Divide1 : Product  Inputs=*/
  Divide2 : Product  Inputs=*/
  Integrator1 : Integrator
  Rate Transition : RateTransition  Commented=through
  Saturation5 : Saturate  UpperLimit=0.0225  LowerLimit=0.01
  Subsystem : Subsystem
  to mm : Gain  Gain=1000
  current : Outport
  wires:
  airgap/1 -> Saturation5/1
  Divide/1 -> Integrator1/1
  Add/1 -> Divide/1
  Integrator1/1 -> Delay1/1, current/1, Delay3/1, Add/2  "current applied"
  2-D Lookup Table/1 -> Divide2/1  "L"
  target current/1 -> Divide1/1
  temperature/1 -> Delay2/1
  Divide1/1 -> Add/1
  Subsystem/1(R) -> Divide2/2, Divide1/2  "R"
  Delay3/1 -> Subsystem/1(Current)
  Delay2/1 -> Subsystem/2(Temperature)
  Divide2/1 -> Divide/2
  Delay1/1 -> 2-D Lookup Table/2
  Rate Transition/1 -> 2-D Lookup Table/1
  Saturation5/1 -> to mm/1
  to mm/1 -> Delay4/1
  Delay4/1 -> Rate Transition/1

== system H8_6GDL_lineal_modelo/HEMS/RL3 ==
  target current : Inport
  airgap : Inport  Port=2
  temperature : Inport  Port=3
  2-D Lookup Table : Lookup_n-D  BreakpointsForDimension1=hems.Airgap  BreakpointsForDimension2=hems.Current(2:110)  Table=hems.Inductance  InternalRulePriority=Speed  RndMeth=Simplest
      settings: InputPortMap=u0,u1
  Add : Sum  Inputs=+-
  Delay{1..4} (4 alike) : Delay  DelayLength=1
  Divide : Product  Inputs=*/
  Divide1 : Product  Inputs=*/
  Divide2 : Product  Inputs=*/
  Integrator1 : Integrator
  Rate Transition : RateTransition  Commented=through
  Saturation5 : Saturate  UpperLimit=0.0225  LowerLimit=0.01
  Subsystem : Subsystem
  to mm : Gain  Gain=1000
  current : Outport
  wires:
  airgap/1 -> Saturation5/1
  Divide/1 -> Integrator1/1
  Add/1 -> Divide/1
  Integrator1/1 -> Delay1/1, current/1, Delay3/1, Add/2  "current applied"
  2-D Lookup Table/1 -> Divide2/1  "L"
  target current/1 -> Divide1/1
  temperature/1 -> Delay2/1
  Divide1/1 -> Add/1
  Subsystem/1(R) -> Divide2/2, Divide1/2  "R"
  Delay3/1 -> Subsystem/1(Current)
  Delay2/1 -> Subsystem/2(Temperature)
  Divide2/1 -> Divide/2
  Delay1/1 -> 2-D Lookup Table/2
  Rate Transition/1 -> 2-D Lookup Table/1
  Saturation5/1 -> to mm/1
  to mm/1 -> Delay4/1
  Delay4/1 -> Rate Transition/1

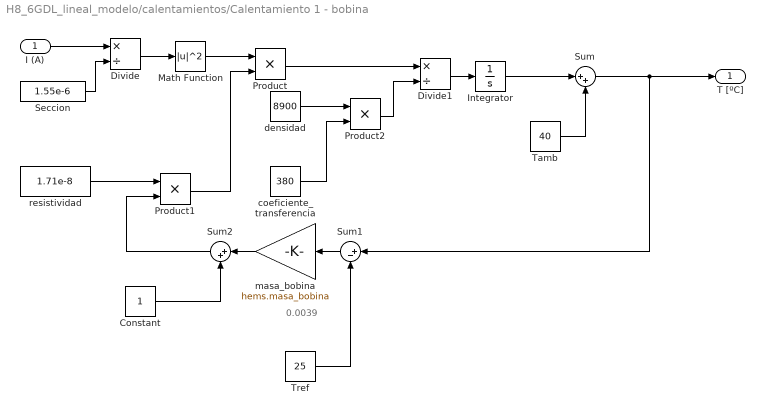
== system H8_6GDL_lineal_modelo/calentamientos/Calentamiento 1 - bobina ==
  note: 0.0039
  I (A) : Inport
  Constant : Constant
  Divide : Product  Inputs=*/
  Divide1 : Product  Inputs=*/
  Integrator : Integrator
  Math Function : Math  Operator=magnitude^2
  Product : Product
  Product1 : Product
  Product2 : Product
  Seccion : Constant  Value=1.55e-6
  Sum : Sum  Inputs=|++
  Sum1 : Sum  Inputs=|+-
  Sum2 : Sum  Inputs=|++
  Tamb : Constant  Value=40
  Tref : Constant  Value=25
  coeficiente_transferencia : Constant  Value=380
  densidad : Constant  Value=8900
  masa_bobina : Gain  Gain=hems.masa_bobina
  resistividad : Constant  Value=1.71e-8
  T [ºC] : Outport
  wires:
  I (A)/1 -> Divide/1
  Seccion/1 -> Divide/2
  Divide/1 -> Math Function/1
  Math Function/1 -> Product/1
  Product/1 -> Divide1/1
  Divide1/1 -> Integrator/1
  Integrator/1 -> Sum/1
  Tamb/1 -> Sum/2
  Sum/1 -> Sum1/1, T [ºC]/1
  Sum1/1 -> masa_bobina/1
  Tref/1 -> Sum1/2
  masa_bobina/1 -> Sum2/1
  Constant/1 -> Sum2/2
  resistividad/1 -> Product1/1
  Sum2/1 -> Product1/2
  Product1/1 -> Product/2
  Product2/1 -> Divide1/2
  densidad/1 -> Product2/1
  coeficiente_transferencia/1 -> Product2/2

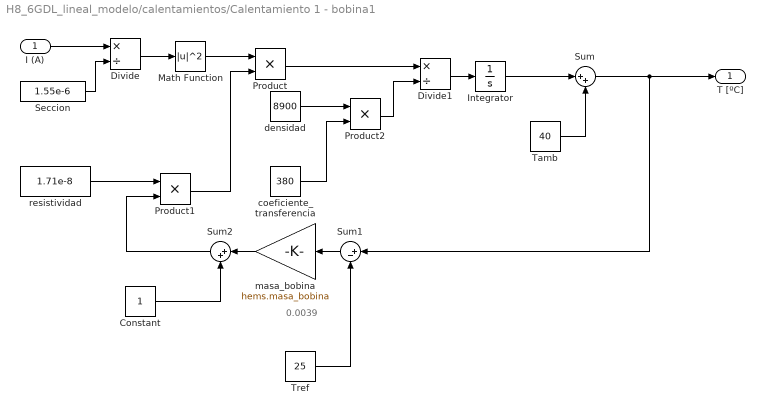
== system H8_6GDL_lineal_modelo/calentamientos/Calentamiento 1 - bobina1 ==
  note: 0.0039
  I (A) : Inport
  Constant : Constant
  Divide : Product  Inputs=*/
  Divide1 : Product  Inputs=*/
  Integrator : Integrator
  Math Function : Math  Operator=magnitude^2
  Product : Product
  Product1 : Product
  Product2 : Product
  Seccion : Constant  Value=1.55e-6
  Sum : Sum  Inputs=|++
  Sum1 : Sum  Inputs=|+-
  Sum2 : Sum  Inputs=|++
  Tamb : Constant  Value=40
  Tref : Constant  Value=25
  coeficiente_transferencia : Constant  Value=380
  densidad : Constant  Value=8900
  masa_bobina : Gain  Gain=hems.masa_bobina
  resistividad : Constant  Value=1.71e-8
  T [ºC] : Outport
  wires:
  I (A)/1 -> Divide/1
  Seccion/1 -> Divide/2
  Divide/1 -> Math Function/1
  Math Function/1 -> Product/1
  Product/1 -> Divide1/1
  Divide1/1 -> Integrator/1
  Integrator/1 -> Sum/1
  Tamb/1 -> Sum/2
  Sum/1 -> Sum1/1, T [ºC]/1
  Sum1/1 -> masa_bobina/1
  Tref/1 -> Sum1/2
  masa_bobina/1 -> Sum2/1
  Constant/1 -> Sum2/2
  resistividad/1 -> Product1/1
  Sum2/1 -> Product1/2
  Product1/1 -> Product/2
  Product2/1 -> Divide1/2
  densidad/1 -> Product2/1
  coeficiente_transferencia/1 -> Product2/2

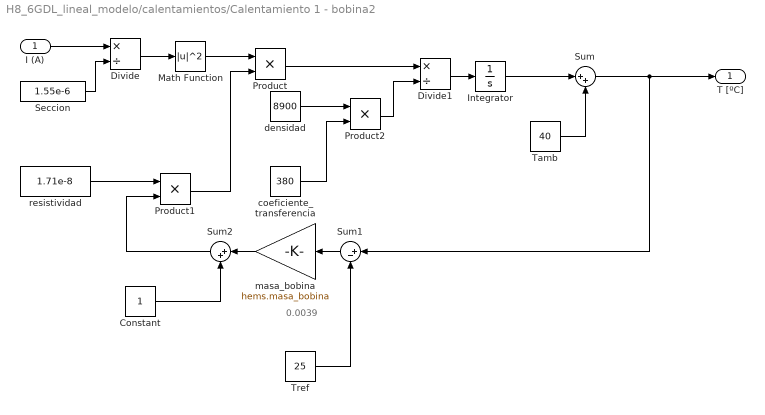
== system H8_6GDL_lineal_modelo/calentamientos/Calentamiento 1 - bobina2 ==
  note: 0.0039
  I (A) : Inport
  Constant : Constant
  Divide : Product  Inputs=*/
  Divide1 : Product  Inputs=*/
  Integrator : Integrator
  Math Function : Math  Operator=magnitude^2
  Product : Product
  Product1 : Product
  Product2 : Product
  Seccion : Constant  Value=1.55e-6
  Sum : Sum  Inputs=|++
  Sum1 : Sum  Inputs=|+-
  Sum2 : Sum  Inputs=|++
  Tamb : Constant  Value=40
  Tref : Constant  Value=25
  coeficiente_transferencia : Constant  Value=380
  densidad : Constant  Value=8900
  masa_bobina : Gain  Gain=hems.masa_bobina
  resistividad : Constant  Value=1.71e-8
  T [ºC] : Outport
  wires:
  I (A)/1 -> Divide/1
  Seccion/1 -> Divide/2
  Divide/1 -> Math Function/1
  Math Function/1 -> Product/1
  Product/1 -> Divide1/1
  Divide1/1 -> Integrator/1
  Integrator/1 -> Sum/1
  Tamb/1 -> Sum/2
  Sum/1 -> Sum1/1, T [ºC]/1
  Sum1/1 -> masa_bobina/1
  Tref/1 -> Sum1/2
  masa_bobina/1 -> Sum2/1
  Constant/1 -> Sum2/2
  resistividad/1 -> Product1/1
  Sum2/1 -> Product1/2
  Product1/1 -> Product/2
  Product2/1 -> Divide1/2
  densidad/1 -> Product2/1
  coeficiente_transferencia/1 -> Product2/2

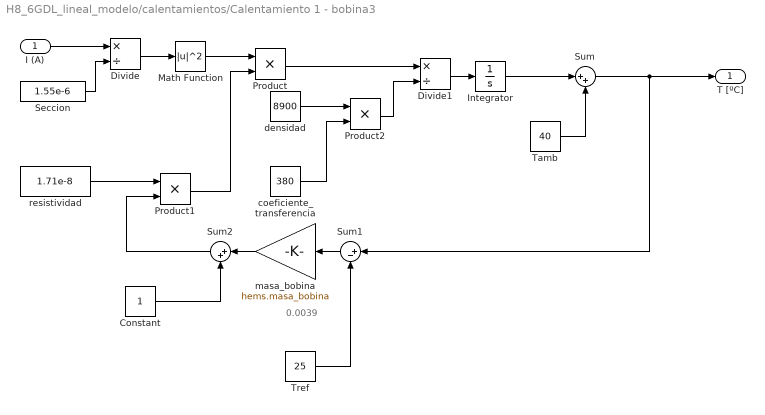
== system H8_6GDL_lineal_modelo/calentamientos/Calentamiento 1 - bobina3 ==
  note: 0.0039
  I (A) : Inport
  Constant : Constant
  Divide : Product  Inputs=*/
  Divide1 : Product  Inputs=*/
  Integrator : Integrator
  Math Function : Math  Operator=magnitude^2
  Product : Product
  Product1 : Product
  Product2 : Product
  Seccion : Constant  Value=1.55e-6
  Sum : Sum  Inputs=|++
  Sum1 : Sum  Inputs=|+-
  Sum2 : Sum  Inputs=|++
  Tamb : Constant  Value=40
  Tref : Constant  Value=25
  coeficiente_transferencia : Constant  Value=380
  densidad : Constant  Value=8900
  masa_bobina : Gain  Gain=hems.masa_bobina
  resistividad : Constant  Value=1.71e-8
  T [ºC] : Outport
  wires:
  I (A)/1 -> Divide/1
  Seccion/1 -> Divide/2
  Divide/1 -> Math Function/1
  Math Function/1 -> Product/1
  Product/1 -> Divide1/1
  Divide1/1 -> Integrator/1
  Integrator/1 -> Sum/1
  Tamb/1 -> Sum/2
  Sum/1 -> Sum1/1, T [ºC]/1
  Sum1/1 -> masa_bobina/1
  Tref/1 -> Sum1/2
  masa_bobina/1 -> Sum2/1
  Constant/1 -> Sum2/2
  resistividad/1 -> Product1/1
  Sum2/1 -> Product1/2
  Product1/1 -> Product/2
  Product2/1 -> Divide1/2
  densidad/1 -> Product2/1
  coeficiente_transferencia/1 -> Product2/2

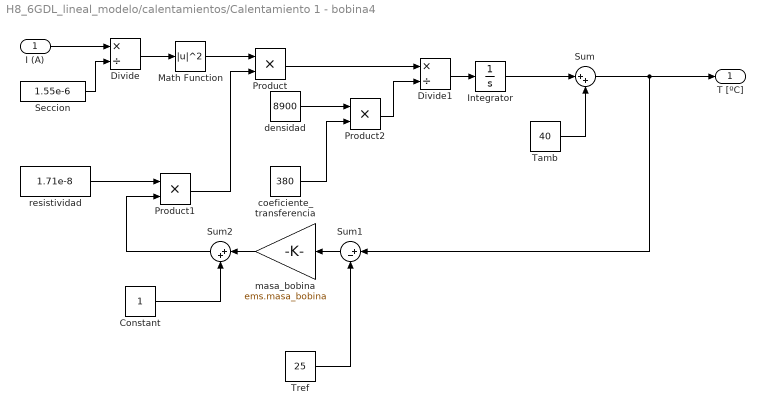
== system H8_6GDL_lineal_modelo/calentamientos/Calentamiento 1 - bobina4 ==
  I (A) : Inport
  Constant : Constant
  Divide : Product  Inputs=*/
  Divide1 : Product  Inputs=*/
  Integrator : Integrator
  Math Function : Math  Operator=magnitude^2
  Product : Product
  Product1 : Product
  Product2 : Product
  Seccion : Constant  Value=1.55e-6
  Sum : Sum  Inputs=|++
  Sum1 : Sum  Inputs=|+-
  Sum2 : Sum  Inputs=|++
  Tamb : Constant  Value=40
  Tref : Constant  Value=25
  coeficiente_transferencia : Constant  Value=380
  densidad : Constant  Value=8900
  masa_bobina : Gain  Gain=ems.masa_bobina
  resistividad : Constant  Value=1.71e-8
  T [ºC] : Outport
  wires:
  I (A)/1 -> Divide/1
  Seccion/1 -> Divide/2
  Divide/1 -> Math Function/1
  Math Function/1 -> Product/1
  Product/1 -> Divide1/1
  Divide1/1 -> Integrator/1
  Integrator/1 -> Sum/1
  Tamb/1 -> Sum/2
  Sum/1 -> Sum1/1, T [ºC]/1
  Sum1/1 -> masa_bobina/1
  Tref/1 -> Sum1/2
  masa_bobina/1 -> Sum2/1
  Constant/1 -> Sum2/2
  resistividad/1 -> Product1/1
  Sum2/1 -> Product1/2
  Product1/1 -> Product/2
  Product2/1 -> Divide1/2
  densidad/1 -> Product2/1
  coeficiente_transferencia/1 -> Product2/2

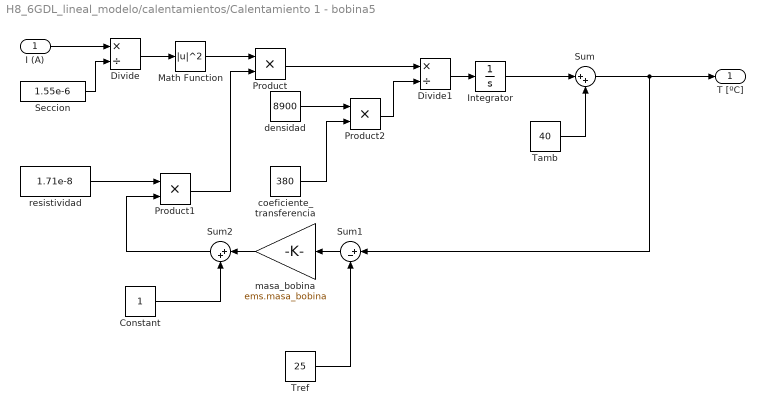
== system H8_6GDL_lineal_modelo/calentamientos/Calentamiento 1 - bobina5 ==
  I (A) : Inport
  Constant : Constant
  Divide : Product  Inputs=*/
  Divide1 : Product  Inputs=*/
  Integrator : Integrator
  Math Function : Math  Operator=magnitude^2
  Product : Product
  Product1 : Product
  Product2 : Product
  Seccion : Constant  Value=1.55e-6
  Sum : Sum  Inputs=|++
  Sum1 : Sum  Inputs=|+-
  Sum2 : Sum  Inputs=|++
  Tamb : Constant  Value=40
  Tref : Constant  Value=25
  coeficiente_transferencia : Constant  Value=380
  densidad : Constant  Value=8900
  masa_bobina : Gain  Gain=ems.masa_bobina
  resistividad : Constant  Value=1.71e-8
  T [ºC] : Outport
  wires:
  I (A)/1 -> Divide/1
  Seccion/1 -> Divide/2
  Divide/1 -> Math Function/1
  Math Function/1 -> Product/1
  Product/1 -> Divide1/1
  Divide1/1 -> Integrator/1
  Integrator/1 -> Sum/1
  Tamb/1 -> Sum/2
  Sum/1 -> Sum1/1, T [ºC]/1
  Sum1/1 -> masa_bobina/1
  Tref/1 -> Sum1/2
  masa_bobina/1 -> Sum2/1
  Constant/1 -> Sum2/2
  resistividad/1 -> Product1/1
  Sum2/1 -> Product1/2
  Product1/1 -> Product/2
  Product2/1 -> Divide1/2
  densidad/1 -> Product2/1
  coeficiente_transferencia/1 -> Product2/2

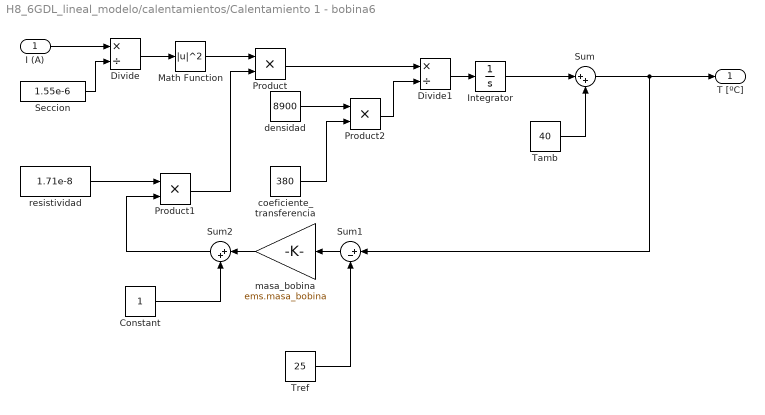
== system H8_6GDL_lineal_modelo/calentamientos/Calentamiento 1 - bobina6 ==
  I (A) : Inport
  Constant : Constant
  Divide : Product  Inputs=*/
  Divide1 : Product  Inputs=*/
  Integrator : Integrator
  Math Function : Math  Operator=magnitude^2
  Product : Product
  Product1 : Product
  Product2 : Product
  Seccion : Constant  Value=1.55e-6
  Sum : Sum  Inputs=|++
  Sum1 : Sum  Inputs=|+-
  Sum2 : Sum  Inputs=|++
  Tamb : Constant  Value=40
  Tref : Constant  Value=25
  coeficiente_transferencia : Constant  Value=380
  densidad : Constant  Value=8900
  masa_bobina : Gain  Gain=ems.masa_bobina
  resistividad : Constant  Value=1.71e-8
  T [ºC] : Outport
  wires:
  I (A)/1 -> Divide/1
  Seccion/1 -> Divide/2
  Divide/1 -> Math Function/1
  Math Function/1 -> Product/1
  Product/1 -> Divide1/1
  Divide1/1 -> Integrator/1
  Integrator/1 -> Sum/1
  Tamb/1 -> Sum/2
  Sum/1 -> Sum1/1, T [ºC]/1
  Sum1/1 -> masa_bobina/1
  Tref/1 -> Sum1/2
  masa_bobina/1 -> Sum2/1
  Constant/1 -> Sum2/2
  resistividad/1 -> Product1/1
  Sum2/1 -> Product1/2
  Product1/1 -> Product/2
  Product2/1 -> Divide1/2
  densidad/1 -> Product2/1
  coeficiente_transferencia/1 -> Product2/2

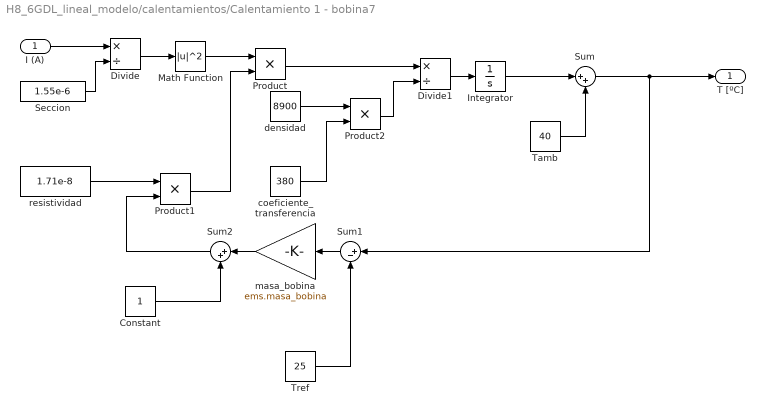
== system H8_6GDL_lineal_modelo/calentamientos/Calentamiento 1 - bobina7 ==
  I (A) : Inport
  Constant : Constant
  Divide : Product  Inputs=*/
  Divide1 : Product  Inputs=*/
  Integrator : Integrator
  Math Function : Math  Operator=magnitude^2
  Product : Product
  Product1 : Product
  Product2 : Product
  Seccion : Constant  Value=1.55e-6
  Sum : Sum  Inputs=|++
  Sum1 : Sum  Inputs=|+-
  Sum2 : Sum  Inputs=|++
  Tamb : Constant  Value=40
  Tref : Constant  Value=25
  coeficiente_transferencia : Constant  Value=380
  densidad : Constant  Value=8900
  masa_bobina : Gain  Gain=ems.masa_bobina
  resistividad : Constant  Value=1.71e-8
  T [ºC] : Outport
  wires:
  I (A)/1 -> Divide/1
  Seccion/1 -> Divide/2
  Divide/1 -> Math Function/1
  Math Function/1 -> Product/1
  Product/1 -> Divide1/1
  Divide1/1 -> Integrator/1
  Integrator/1 -> Sum/1
  Tamb/1 -> Sum/2
  Sum/1 -> Sum1/1, T [ºC]/1
  Sum1/1 -> masa_bobina/1
  Tref/1 -> Sum1/2
  masa_bobina/1 -> Sum2/1
  Constant/1 -> Sum2/2
  resistividad/1 -> Product1/1
  Sum2/1 -> Product1/2
  Product1/1 -> Product/2
  Product2/1 -> Divide1/2
  densidad/1 -> Product2/1
  coeficiente_transferencia/1 -> Product2/2

== system H8_6GDL_lineal_modelo/Control/state space control/Moving Average Filter ==
  input : Inport
  Delay : Delay  DelayLength=M  SampleTime=fs
  Delay1 : Delay  DelayLength=1  SampleTime=fs
  Gain : Gain  Gain=1/M
  Sum : Sum  Inputs=|+-
  Sum1 : Sum  Inputs=|++
  output : Outport
  wires:
  input/1 -> Delay/1, Sum/1
  Delay/1 -> Sum/2
  Sum/1 -> Sum1/1
  Sum1/1 -> Delay1/1, Gain/1
  Delay1/1 -> Sum1/2
  Gain/1 -> output/1

== system H8_6GDL_lineal_modelo/Control/state space control/Moving Average Filter1 ==
  input : Inport
  Delay : Delay  DelayLength=M  SampleTime=fs
  Delay1 : Delay  DelayLength=1  SampleTime=fs
  Gain : Gain  Gain=1/M
  Sum : Sum  Inputs=|+-
  Sum1 : Sum  Inputs=|++
  output : Outport
  wires:
  input/1 -> Delay/1, Sum/1
  Delay/1 -> Sum/2
  Sum/1 -> Sum1/1
  Sum1/1 -> Delay1/1, Gain/1
  Delay1/1 -> Sum1/2
  Gain/1 -> output/1

== system H8_6GDL_lineal_modelo/Control/state space control/Moving Average Filter2 ==
  input : Inport
  Delay : Delay  DelayLength=M  SampleTime=fs
  Delay1 : Delay  DelayLength=1  SampleTime=fs
  Gain : Gain  Gain=1/M
  Sum : Sum  Inputs=|+-
  Sum1 : Sum  Inputs=|++
  output : Outport
  wires:
  input/1 -> Delay/1, Sum/1
  Delay/1 -> Sum/2
  Sum/1 -> Sum1/1
  Sum1/1 -> Delay1/1, Gain/1
  Delay1/1 -> Sum1/2
  Gain/1 -> output/1

== system H8_6GDL_lineal_modelo/Control/state space control/Moving Average Filter3 ==
  input : Inport
  Delay : Delay  DelayLength=M  SampleTime=fs
  Delay1 : Delay  DelayLength=1  SampleTime=fs
  Gain : Gain  Gain=1/M
  Sum : Sum  Inputs=|+-
  Sum1 : Sum  Inputs=|++
  output : Outport
  wires:
  input/1 -> Delay/1, Sum/1
  Delay/1 -> Sum/2
  Sum/1 -> Sum1/1
  Sum1/1 -> Delay1/1, Gain/1
  Delay1/1 -> Sum1/2
  Gain/1 -> output/1

== system H8_6GDL_lineal_modelo/Control/state space control/Moving Average Filter4 ==
  input : Inport
  Delay : Delay  DelayLength=M  SampleTime=fs
  Delay1 : Delay  DelayLength=1  SampleTime=fs
  Gain : Gain  Gain=1/M
  Sum : Sum  Inputs=|+-
  Sum1 : Sum  Inputs=|++
  output : Outport
  wires:
  input/1 -> Delay/1, Sum/1
  Delay/1 -> Sum/2
  Sum/1 -> Sum1/1
  Sum1/1 -> Delay1/1, Gain/1
  Delay1/1 -> Sum1/2
  Gain/1 -> output/1

== system H8_6GDL_lineal_modelo/EMS/RL/Subsystem ==
  Current : Inport
  Temperature : Inport  Port=2
  Resistance : Constant  Value=ems.Resistance
  R : Outport
  wires:
  Resistance/1 -> R/1

== system H8_6GDL_lineal_modelo/EMS/RL1/Subsystem ==
  Current : Inport
  Temperature : Inport  Port=2
  Resistance : Constant  Value=ems.Resistance
  R : Outport
  wires:
  Resistance/1 -> R/1

== system H8_6GDL_lineal_modelo/EMS/RL2/Subsystem ==
  Current : Inport
  Temperature : Inport  Port=2
  Resistance : Constant  Value=ems.Resistance
  R : Outport
  wires:
  Resistance/1 -> R/1

== system H8_6GDL_lineal_modelo/EMS/RL3/Subsystem ==
  Current : Inport
  Temperature : Inport  Port=2
  Resistance : Constant  Value=ems.Resistance
  R : Outport
  wires:
  Resistance/1 -> R/1

== system H8_6GDL_lineal_modelo/HEMS/RL/Subsystem ==
  Current : Inport
  Temperature : Inport  Port=2
  Resistance : Constant  Value=hems.Resistance
  R : Outport
  wires:
  Resistance/1 -> R/1

== system H8_6GDL_lineal_modelo/HEMS/RL1/Subsystem ==
  Current : Inport
  Temperature : Inport  Port=2
  Resistance : Constant  Value=hems.Resistance
  R : Outport
  wires:
  Resistance/1 -> R/1

== system H8_6GDL_lineal_modelo/HEMS/RL2/Subsystem ==
  Current : Inport
  Temperature : Inport  Port=2
  Resistance : Constant  Value=hems.Resistance
  R : Outport
  wires:
  Resistance/1 -> R/1

== system H8_6GDL_lineal_modelo/HEMS/RL3/Subsystem ==
  Current : Inport
  Temperature : Inport  Port=2
  Resistance : Constant  Value=hems.Resistance
  R : Outport
  wires:
  Resistance/1 -> R/1
